simulink model "PCM_Encoder"  (R2021a)
settings: Solver=VariableStepAuto  StartTime=0.0  StopTime=1e-3 - eps  FixedStep=1/(48e-7)  MaxStep=1e-5  RelTol=1e-3
model workspace (MAT data in the model file):
  BitDepth = 4
  DecimationFactor = 3
  DemoMode = 1
  Dithering = 0
  FirDenominatorCoefficients = [1 1]
  FirNumeratorCoefficients = [1 1]
  IsLinear = 1
  LowerSaturation = -2.5
  SampleRate = 48000
  UpperSaturation = 2.5
libraries: simulink x5, commsrccod2 x1
settings Model: OrderedModelArguments=off  Creator=james  LastModifiedBy=james

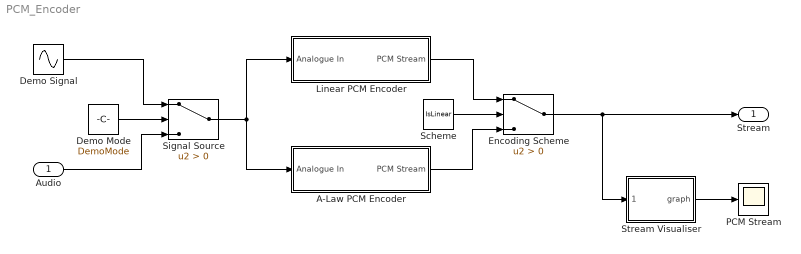
== system PCM_Encoder ==
  Audio : Inport  SampleTime=1/SampleRate
  A-Law PCM Encoder : Subsystem
  Demo Mode : Constant  Value=DemoMode
  Demo Signal : Sin  Amplitude=2.4  Frequency=2*pi*2000  SampleTime=1/SampleRate
  Encoding Scheme : Switch  Criteria=u2 > Threshold
  Linear PCM Encoder : Subsystem
  PCM Stream : Scope
  Scheme : Constant  Value=IsLinear
  Signal Source : Switch  Criteria=u2 > Threshold
  Stream Visualiser : Subsystem
  Stream : Outport
  wires:
  Stream Visualiser/1(graph) -> PCM Stream/1
  Demo Mode/1 -> Signal Source/2
  Signal Source/1 -> A-Law PCM Encoder/1(Analogue In), Linear PCM Encoder/1(Analogue In)
  Encoding Scheme/1 -> Stream Visualiser/1(uint4_t), Stream/1
  Scheme/1 -> Encoding Scheme/2
  Linear PCM Encoder/1(PCM Stream) -> Encoding Scheme/1
  A-Law PCM Encoder/1(PCM Stream) -> Encoding Scheme/3
  Demo Signal/1 -> Signal Source/1
  Audio/1 -> Signal Source/3

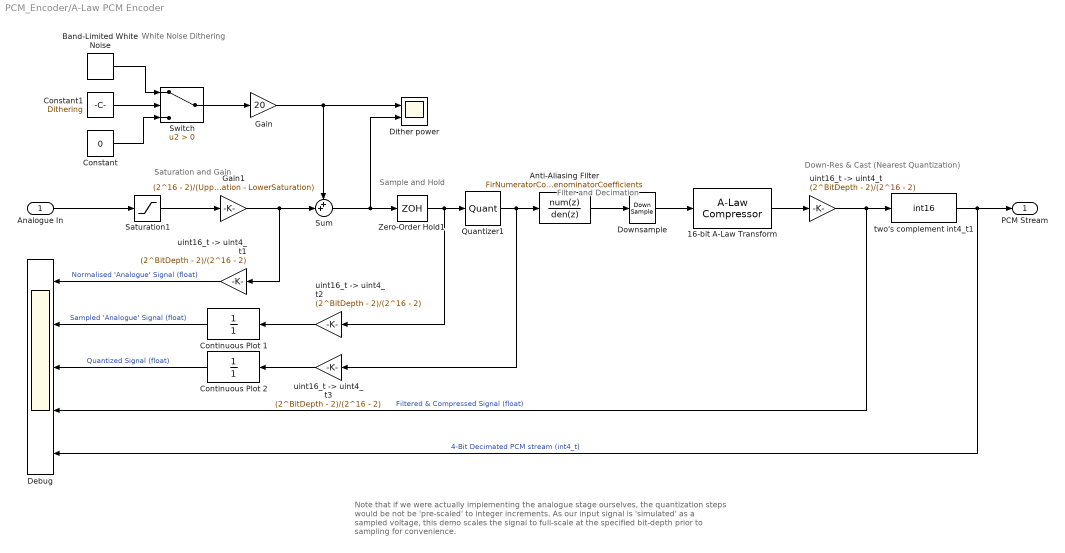
== system PCM_Encoder/A-Law PCM Encoder ==
  note: Filter and Decimation
  note: Note that if we were actually implementing the analogue stage ourselves, the quantization steps would be not be 'pre-scaled' to integer increments. As our input signal is 'simulated' as a sampled voltage, this demo scales the signal to full-scale at the specified bit-depth prior to sampling for convenience.
  note: Down-Res & Cast (Nearest Quantization)
  note: Sample and Hold
  note: Saturation and Gain
  note: White Noise Dithering
  Analogue In : Inport
  16-bit A-Law Transform : commsrccod2/A-Law Compressor  A=87.6  V=(2^16 - 1)/2
      settings: SourceProductBaseCode=CM
  Anti-Aliasing Filter : DiscreteTransferFcn  Numerator=FirNumeratorCoefficients  Denominator=FirDenominatorCoefficients
  Band-Limited White Noise : simulink/Sources/Band-Limited White Noise  Cov=[0.1]  Ts=1/SampleRate  seed=[23341]
  Constant : Constant  Value=0  SampleTime=1/SampleRate
  Constant1 : Constant  Value=Dithering
  Continuous Plot 1 : TransferFcn  Denominator=[1]  ContinuousStateAttributes="''Continuous\""
  Continuous Plot 2 : TransferFcn  Denominator=[1]  ContinuousStateAttributes="''Continuous\""
  Debug : Scope  NumInputPorts=5
  Dither power : Scope  NumInputPorts=2
  Downsample : DownSample  N=DecimationFactor  RateOptions=Allow multirate processing
  Gain : Gain  Gain=20
  Gain1 : Gain  Gain=(2^16 - 2)/(UpperSaturation - LowerSaturation)
  Quantizer1 : Quantizer  QuantizationInterval=1  LinearizeAsGain=off
  Saturation1 : Saturate  UpperLimit=2.5  LowerLimit=-2.5
  Sum : Sum  Inputs=++|
  Switch : Switch  Criteria=u2 > Threshold
  Zero-Order Hold1 : ZeroOrderHold  SampleTime=1/SampleRate
  two's complement int4_t1 : DataTypeConversion  OutDataTypeStr=int16  RndMeth=Nearest
  uint16_t -> uint4_t{,1..3} (4 alike) : Gain  Gain=(2^BitDepth - 2)/(2^16 - 2)
  PCM Stream : Outport
  wires:
  Continuous Plot 1/1 -> Debug/2  "Sampled 'Analogue' Signal (float)"
  Continuous Plot 2/1 -> Debug/3  "Quantized Signal (float)"
  Anti-Aliasing Filter/1 -> Downsample/1
  Zero-Order Hold1/1 -> Quantizer1/1, "uint16_t -> uint4_t2"/1
  Gain1/1 -> Sum/2, "uint16_t -> uint4_t1"/1
  Analogue In/1 -> Saturation1/1
  Saturation1/1 -> Gain1/1
  two's complement int4_t1/1 -> Debug/5, PCM Stream/1  "4-Bit Decimated PCM stream (int4_t)"
  Quantizer1/1 -> Anti-Aliasing Filter/1, "uint16_t -> uint4_t3"/1
  16-bit A-Law Transform/1 -> "uint16_t -> uint4_t"/1
  Downsample/1 -> 16-bit A-Law Transform/1
  "uint16_t -> uint4_t1"/1 -> Debug/1  "Normalised 'Analogue' Signal (float)"
  "uint16_t -> uint4_t2"/1 -> Continuous Plot 1/1
  "uint16_t -> uint4_t3"/1 -> Continuous Plot 2/1
  "uint16_t -> uint4_t"/1 -> Debug/4, two's complement int4_t1/1  "Filtered & Compressed Signal (float)"
  Constant1/1 -> Switch/2
  Constant/1 -> Switch/3
  Switch/1 -> Gain/1
  Sum/1 -> Zero-Order Hold1/1, Dither power/2
  Gain/1 -> Dither power/1, Sum/1
  Band-Limited White Noise/1 -> Switch/1

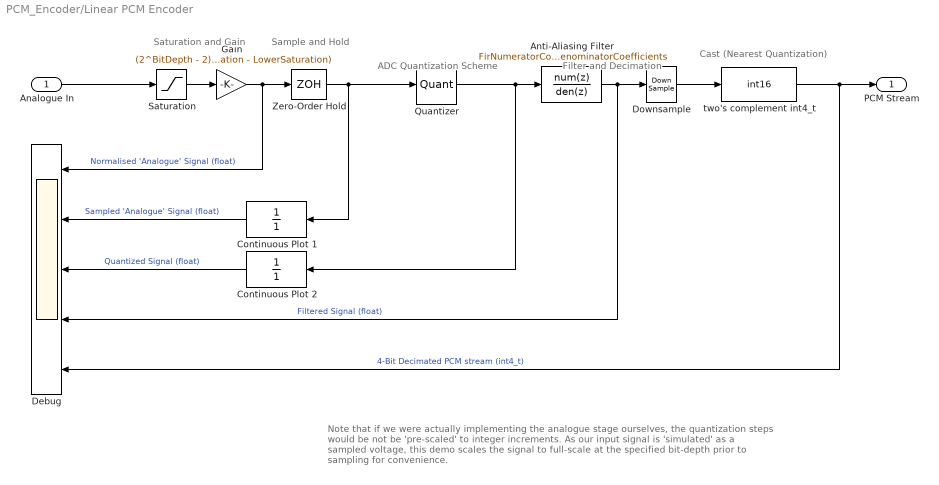
== system PCM_Encoder/Linear PCM Encoder ==
  note: Note that if we were actually implementing the analogue stage ourselves, the quantization steps would be not be 'pre-scaled' to integer increments. As our input signal is 'simulated' as a sampled voltage, this demo scales the signal to full-scale at the specified bit-depth prior to sampling for convenience.
  note: Cast (Nearest Quantization)
  note: Saturation and Gain
  note: Filter and Decimation
  note: Sample and Hold
  note: ADC Quantization Scheme
  Analogue In : Inport
  Anti-Aliasing Filter : DiscreteTransferFcn  Numerator=FirNumeratorCoefficients  Denominator=FirDenominatorCoefficients
  Continuous Plot 1 : TransferFcn  Denominator=[1]  ContinuousStateAttributes="''Continuous\""
  Continuous Plot 2 : TransferFcn  Denominator=[1]  ContinuousStateAttributes="''Continuous\""
  Debug : Scope  NumInputPorts=5
  Downsample : DownSample  N=DecimationFactor  RateOptions=Allow multirate processing
  Gain : Gain  Gain=(2^BitDepth - 2)/(UpperSaturation - LowerSaturation)
  Quantizer : Quantizer  QuantizationInterval=1  LinearizeAsGain=off
  Saturation : Saturate  UpperLimit=2.5  LowerLimit=-2.5
  Zero-Order Hold : ZeroOrderHold  SampleTime=1/SampleRate
  two's complement int4_t : DataTypeConversion  OutDataTypeStr=int16  RndMeth=Nearest
  PCM Stream : Outport
  wires:
  Saturation/1 -> Gain/1
  Gain/1 -> Debug/1, Zero-Order Hold/1  "Normalised 'Analogue' Signal (float)"
  Zero-Order Hold/1 -> Quantizer/1, Continuous Plot 1/1
  two's complement int4_t/1 -> Debug/5, PCM Stream/1  "4-Bit Decimated PCM stream (int4_t)"
  Downsample/1 -> two's complement int4_t/1
  Anti-Aliasing Filter/1 -> Debug/4, Downsample/1  "Filtered Signal (float)"
  Quantizer/1 -> Anti-Aliasing Filter/1, Continuous Plot 2/1
  Continuous Plot 2/1 -> Debug/3  "Quantized Signal (float)"
  Continuous Plot 1/1 -> Debug/2  "Sampled 'Analogue' Signal (float)"
  Analogue In/1 -> Saturation/1

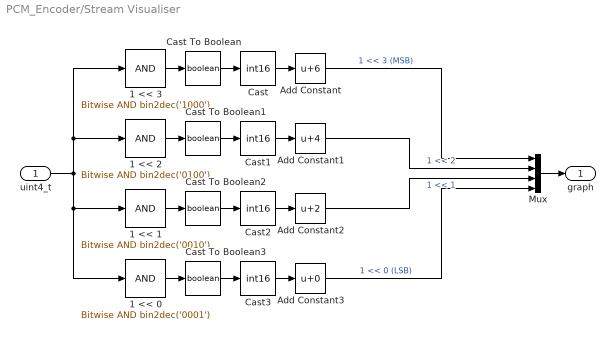
== system PCM_Encoder/Stream Visualiser ==
  uint4_t : Inport
  1 << 0 : simulink/Logic and Bit Operations/Bitwise Operator  logicop=AND  UseBitMask=on  BitMask=bin2dec('0001')  BitMaskRealWorld=Stored Integer
  1 << 1 : simulink/Logic and Bit Operations/Bitwise Operator  logicop=AND  UseBitMask=on  BitMask=bin2dec('0010')  BitMaskRealWorld=Stored Integer
  1 << 2 : simulink/Logic and Bit Operations/Bitwise Operator  logicop=AND  UseBitMask=on  BitMask=bin2dec('0100')  BitMaskRealWorld=Stored Integer
  1 << 3 : simulink/Logic and Bit Operations/Bitwise Operator  logicop=AND  UseBitMask=on  BitMask=bin2dec('1000')  BitMaskRealWorld=Stored Integer
  Add Constant : Bias  Bias=6
  Add Constant1 : Bias  Bias=4
  Add Constant2 : Bias  Bias=2
  Add Constant3 : Bias
  Cast{,1..3} (4 alike) : DataTypeConversion  OutDataTypeStr=int16
  Cast To Boolean{,1..3} (4 alike) : DataTypeConversion  OutDataTypeStr=boolean
  Mux : Mux
  graph : Outport
  wires:
  uint4_t/1 -> 1 << 0/1, 1 << 1/1, 1 << 3/1, 1 << 2/1
  Mux/1 -> graph/1
  1 << 2/1 -> Cast To Boolean1/1
  1 << 1/1 -> Cast To Boolean2/1
  1 << 0/1 -> Cast To Boolean3/1
  1 << 3/1 -> Cast To Boolean/1
  Cast To Boolean/1 -> Cast/1
  Cast/1 -> Add Constant/1
  Add Constant/1 -> Mux/1  "1 << 3 (MSB)"
  Add Constant1/1 -> Mux/2  "1 << 2"
  Cast1/1 -> Add Constant1/1
  Cast To Boolean1/1 -> Cast1/1
  Add Constant2/1 -> Mux/3  "1 << 1"
  Cast To Boolean2/1 -> Cast2/1
  Cast2/1 -> Add Constant2/1
  Cast3/1 -> Add Constant3/1
  Add Constant3/1 -> Mux/4  "1 << 0 (LSB)"
  Cast To Boolean3/1 -> Cast3/1
